simulink model "Channelizer_orig"  (R2026a)
settings: Solver=VariableStepAuto  StopTime=1e-5
InitFcn:
  | init;
values from neighbouring files (symbols this model uses):
  ch0_en = 0    [channelizer_demo_init.m]    (also in init.m)
  ch0_qam = 0    [channelizer_demo_init.m]    (also in init.m)
  ch0_swp = 0    [channelizer_demo_init.m]    (also in init.m)
  ch10_en = 0    [channelizer_demo_init.m]    (also in init.m)
  ch10_qam = 0    [channelizer_demo_init.m]    (also in init.m)
  ch10_swp = 0    [channelizer_demo_init.m]    (also in init.m)
  ch11_en = 0    [channelizer_demo_init.m]    (also in init.m)
  ch11_qam = 0    [channelizer_demo_init.m]    (also in init.m)
  ch11_swp = 0    [channelizer_demo_init.m]    (also in init.m)
  ch12_en = 0    [channelizer_demo_init.m]    (also in init.m)
  ch12_qam = 0    [channelizer_demo_init.m]    (also in init.m)
  ch12_swp = 0    [channelizer_demo_init.m]    (also in init.m)
  ch13_en = 0    [channelizer_demo_init.m]    (also in init.m)
  ch13_qam = 0    [channelizer_demo_init.m]    (also in init.m)
  ch13_swp = 0    [channelizer_demo_init.m]    (also in init.m)
  ch14_en = 0    [channelizer_demo_init.m]    (also in init.m)
  ch14_qam = 0    [channelizer_demo_init.m]    (also in init.m)
  ch14_swp = 0    [channelizer_demo_init.m]    (also in init.m)
  ch15_en = 0    [channelizer_demo_init.m]    (also in init.m)
  ch15_qam = 0    [channelizer_demo_init.m]    (also in init.m)
  ch15_swp = 0    [channelizer_demo_init.m]    (also in init.m)
  ch1_en = 1    [channelizer_demo_init.m]    (also in init.m)
  ch1_qam = 0    [channelizer_demo_init.m]    (also in init.m)
  ch1_swp = 0    [channelizer_demo_init.m]    (also in init.m)
  ch2_en = 1    [channelizer_demo_init.m]    (also in init.m)
  ch2_qam = 0    [channelizer_demo_init.m]    (also in init.m)
  ch2_swp = 0    [channelizer_demo_init.m]    (also in init.m)
  ch3_en = 0    [channelizer_demo_init.m]    (also in init.m)
  ch3_qam = 0    [channelizer_demo_init.m]    (also in init.m)
  ch3_swp = 0    [channelizer_demo_init.m]    (also in init.m)
  ch4_en = 0    [channelizer_demo_init.m]    (also in init.m)
  ch4_qam = 0    [channelizer_demo_init.m]    (also in init.m)
  ch4_swp = 0    [channelizer_demo_init.m]    (also in init.m)
  ch5_en = 1    [channelizer_demo_init.m]    (also in init.m)
  ch5_qam = 1    [channelizer_demo_init.m]    (also in init.m)
  ch5_swp = 0    [channelizer_demo_init.m]    (also in init.m)
  ch6_en = 1    [channelizer_demo_init.m]    (also in init.m)
  ch6_qam = 1    [channelizer_demo_init.m]    (also in init.m)
  ch6_swp = 0    [channelizer_demo_init.m]    (also in init.m)
  ch7_en = 0    [channelizer_demo_init.m]    (also in init.m)
  ch7_qam = 0    [channelizer_demo_init.m]    (also in init.m)
  ch7_swp = 0    [channelizer_demo_init.m]    (also in init.m)
  ch8_en = 0    [channelizer_demo_init.m]    (also in init.m)
  ch8_qam = 0    [channelizer_demo_init.m]    (also in init.m)
  ch8_swp = 0    [channelizer_demo_init.m]    (also in init.m)
  ch9_en = 0    [channelizer_demo_init.m]    (also in init.m)
  ch9_qam = 0    [channelizer_demo_init.m]    (also in init.m)
  ch9_swp = 0    [channelizer_demo_init.m]    (also in init.m)
  ch_filt_coef = 28 * ch_filt_coef / sum(ch_filt_coef(:))    [init.m]
  N = 2*1024    (= 2048)    [hil.m]    (also in init.m = 256)
  nvar = 0.01    [init.m]
  randph = 2*pi*rand(16,1)    [init.m]
  spec1_ch = 1    [channelizer_demo_init.m]    (also in init.m)
  spec2_ch = 2    [channelizer_demo_init.m]    (also in init.m)
  spec3_ch = 5    [channelizer_demo_init.m]    (also in init.m)
  spec4_ch = 6    [channelizer_demo_init.m]    (also in init.m)
  swp_rate0 = 0    [channelizer_demo_init.m]    (also in init.m)
  swp_rate1 = 0    [channelizer_demo_init.m]    (also in init.m)
  swp_rate10 = 0    [channelizer_demo_init.m]    (also in init.m)
  swp_rate11 = 0    [channelizer_demo_init.m]    (also in init.m)
  swp_rate12 = 0    [channelizer_demo_init.m]    (also in init.m)
  swp_rate13 = 0    [channelizer_demo_init.m]    (also in init.m)
  swp_rate14 = 0    [channelizer_demo_init.m]    (also in init.m)
  swp_rate15 = 0    [channelizer_demo_init.m]    (also in init.m)
  swp_rate2 = 0    [channelizer_demo_init.m]    (also in init.m)
  swp_rate3 = 0    [channelizer_demo_init.m]    (also in init.m)
  swp_rate4 = 0    [channelizer_demo_init.m]    (also in init.m)
  swp_rate5 = 0    [channelizer_demo_init.m]    (also in init.m)
  swp_rate6 = 0    [channelizer_demo_init.m]    (also in init.m)
  swp_rate7 = 0    [channelizer_demo_init.m]    (also in init.m)
  swp_rate8 = 0    [channelizer_demo_init.m]    (also in init.m)
  swp_rate9 = 0    [channelizer_demo_init.m]    (also in init.m)
  Ts = 16*(7/4)/8.75e9    (= 3.2e-09)    [init.m]
undefined symbols (not defined in the file or in its folder): Asymmetric, Channelizer, DUT_SSR, jsin, S, vsva2197, xcvc1902
libraries: aieUtilities x20, aieBasic x7, hlsBasic x4, aieDSP x2, vmcUtilities x1
(part 3 of 3)

== system Channelizer_orig/Wideband_Signal/Subsystem5 ==
  swp_en : Inport
  chan_fc : Inport  Port=2
  qam_sym : Inport  Port=3
  qam_en : Inport  Port=4
  chan_en : EnablePort
  Add{1..4} (4 alike) : Sum
  Constant : Constant  Value=complex(ones(28*N,1))  SampleTime=-1
  Constant1 : Constant  Value=complex(zeros(N,27))  VectorParams1D=off  SampleTime=-1
  Constant2 : Constant  Value=(1:28*N)'  SampleTime=-1
  Constant3 : Constant  Value=(1:28*N)'  SampleTime=-1
  Constant4 : Constant  Value=2^32  SampleTime=-1
  Constant5 : Constant  Value=zeros(28*N,1)  SampleTime=-1
  Constant6 : Constant  Value=randph(5)  SampleTime=-1
  Constant7 : Constant  Value=2^32  SampleTime=-1
  Delay1 : Delay  DelayLength=1  InitialCondition=(0:28*N-1)'
  Delay2 : Delay  DelayLength=1  InitialCondition=(1:28*N)'  ExternalReset=Falling  ShowEnablePort=on
      settings: InputPortMap=u0,e6,r5
  Discrete FIR Filter : DiscreteFir  Coefficients=ch_filt_coef  InputProcessing=Columns as channels (frame based)
  Gain1 : Gain  Gain=2*pi  OutDataTypeStr=double
  Gain7 : Gain  Gain=1e-7*swp_rate4  ParamDataTypeStr=double  OutDataTypeStr=double  SaturateOnIntegerOverflow=on
  Gain8 : Gain  Gain=1/16  OutDataTypeStr=double
  Mod : Math  Operator=mod
  Mod1 : Math  Operator=mod
  NOT : Logic  Operator=NOT  IconShape=distinctive  AllPortsSameDT=off  OutDataTypeStr=boolean
  Product : Product
  Product1 : Product
  Product2 : Product
  Reshape : Reshape
  Selector1 : Selector  InputPortWidth=28*N  IndexOptions=Index vector (dialog)  Indices=28*N  OutputSizes=1
  Selector2 : Selector  InputPortWidth=28*N  IndexOptions=Index vector (dialog)  Indices=28*N  OutputSizes=1
  Switch : Switch  Criteria=u2 > Threshold  SaturateOnIntegerOverflow=off  InputSameDT=off
  Switch1 : Switch  Criteria=u2 > Threshold  SaturateOnIntegerOverflow=off  InputSameDT=off
  Transpose : Math  Operator=transpose
  Trigonometric Function : Trigonometry  Operator=cos + jsin
  Vector Concatenate : Concatenate  Mode=Multidimensional array  ConcatenateDimension=2
  chan_out : Outport  OutputWhenDisabled=reset  InitialOutput=zeros(28*N,1)
  wires:
  Product/1 -> chan_out/1
  Switch/1 -> Product/2
  Discrete FIR Filter/1 -> Switch/1
  qam_en/1 -> Switch/2
  Constant/1 -> Switch/3
  Vector Concatenate/1 -> Transpose/1
  qam_sym/1 -> Vector Concatenate/1
  Constant1/1 -> Vector Concatenate/2
  Transpose/1 -> Reshape/1
  Reshape/1 -> Discrete FIR Filter/1
  Delay1/1 -> Product1/1, Selector1/1
  Selector1/1 -> Add3/1
  Constant3/1 -> Add3/2
  Mod/1 -> Delay1/1
  Add3/1 -> Mod/1
  Constant4/1 -> Mod/2
  Constant6/1 -> Add4/1
  Trigonometric Function/1 -> Product/1
  Add4/1 -> Trigonometric Function/1
  chan_fc/1 -> Gain8/1
  Gain8/1 -> Product1/2
  Gain1/1 -> Add4/2
  swp_en/1 -> NOT/1, Delay2/2, Switch1/2
  Constant5/1 -> Switch1/3
  Product2/1 -> Gain7/1
  Gain7/1 -> Switch1/1
  Switch1/1 -> Add1/1
  Product1/1 -> Add1/2
  Add1/1 -> Gain1/1
  Mod1/1 -> Delay2/1
  Constant2/1 -> Add2/2
  Selector2/1 -> Add2/1
  Delay2/1 -> Product2/1, Selector2/1, Product2/2
  Add2/1 -> Mod1/1
  Constant7/1 -> Mod1/2
  NOT/1 -> Delay2/3

== system Channelizer_orig/Wideband_Signal/Subsystem6 ==
  swp_en : Inport
  chan_fc : Inport  Port=2
  qam_sym : Inport  Port=3
  qam_en : Inport  Port=4
  chan_en : EnablePort
  Add{1..4} (4 alike) : Sum
  Constant : Constant  Value=complex(ones(28*N,1))  SampleTime=-1
  Constant1 : Constant  Value=complex(zeros(N,27))  VectorParams1D=off  SampleTime=-1
  Constant2 : Constant  Value=(1:28*N)'  SampleTime=-1
  Constant3 : Constant  Value=(1:28*N)'  SampleTime=-1
  Constant4 : Constant  Value=2^32  SampleTime=-1
  Constant5 : Constant  Value=zeros(28*N,1)  SampleTime=-1
  Constant6 : Constant  Value=randph(6)  SampleTime=-1
  Constant7 : Constant  Value=2^32  SampleTime=-1
  Delay1 : Delay  DelayLength=1  InitialCondition=(0:28*N-1)'
  Delay2 : Delay  DelayLength=1  InitialCondition=(1:28*N)'  ExternalReset=Falling  ShowEnablePort=on
      settings: InputPortMap=u0,e6,r5
  Discrete FIR Filter : DiscreteFir  Coefficients=ch_filt_coef  InputProcessing=Columns as channels (frame based)
  Gain1 : Gain  Gain=2*pi  OutDataTypeStr=double
  Gain7 : Gain  Gain=1e-7*swp_rate5  ParamDataTypeStr=double  OutDataTypeStr=double  SaturateOnIntegerOverflow=on
  Gain8 : Gain  Gain=1/16  OutDataTypeStr=double
  Mod : Math  Operator=mod
  Mod1 : Math  Operator=mod
  NOT : Logic  Operator=NOT  IconShape=distinctive  AllPortsSameDT=off  OutDataTypeStr=boolean
  Product : Product
  Product1 : Product
  Product2 : Product
  Reshape : Reshape
  Selector1 : Selector  InputPortWidth=28*N  IndexOptions=Index vector (dialog)  Indices=28*N  OutputSizes=1
  Selector2 : Selector  InputPortWidth=28*N  IndexOptions=Index vector (dialog)  Indices=28*N  OutputSizes=1
  Switch : Switch  Criteria=u2 > Threshold  SaturateOnIntegerOverflow=off  InputSameDT=off
  Switch1 : Switch  Criteria=u2 > Threshold  SaturateOnIntegerOverflow=off  InputSameDT=off
  Transpose : Math  Operator=transpose
  Trigonometric Function : Trigonometry  Operator=cos + jsin
  Vector Concatenate : Concatenate  Mode=Multidimensional array  ConcatenateDimension=2
  chan_out : Outport  OutputWhenDisabled=reset  InitialOutput=zeros(28*N,1)
  wires:
  Product/1 -> chan_out/1
  Switch/1 -> Product/2
  Discrete FIR Filter/1 -> Switch/1
  qam_en/1 -> Switch/2
  Constant/1 -> Switch/3
  Vector Concatenate/1 -> Transpose/1
  qam_sym/1 -> Vector Concatenate/1
  Constant1/1 -> Vector Concatenate/2
  Transpose/1 -> Reshape/1
  Reshape/1 -> Discrete FIR Filter/1
  Delay1/1 -> Product1/1, Selector1/1
  Selector1/1 -> Add3/1
  Constant3/1 -> Add3/2
  Mod/1 -> Delay1/1
  Add3/1 -> Mod/1
  Constant4/1 -> Mod/2
  Constant6/1 -> Add4/1
  Trigonometric Function/1 -> Product/1
  Add4/1 -> Trigonometric Function/1
  chan_fc/1 -> Gain8/1
  Gain8/1 -> Product1/2
  Gain1/1 -> Add4/2
  swp_en/1 -> NOT/1, Delay2/2, Switch1/2
  Constant5/1 -> Switch1/3
  Product2/1 -> Gain7/1
  Gain7/1 -> Switch1/1
  Switch1/1 -> Add1/1
  Product1/1 -> Add1/2
  Add1/1 -> Gain1/1
  Mod1/1 -> Delay2/1
  Constant2/1 -> Add2/2
  Selector2/1 -> Add2/1
  Delay2/1 -> Product2/1, Selector2/1, Product2/2
  Add2/1 -> Mod1/1
  Constant7/1 -> Mod1/2
  NOT/1 -> Delay2/3

== system Channelizer_orig/Wideband_Signal/Subsystem7 ==
  swp_en : Inport
  chan_fc : Inport  Port=2
  qam_sym : Inport  Port=3
  qam_en : Inport  Port=4
  chan_en : EnablePort
  Add{1..4} (4 alike) : Sum
  Constant : Constant  Value=complex(ones(28*N,1))  SampleTime=-1
  Constant1 : Constant  Value=complex(zeros(N,27))  VectorParams1D=off  SampleTime=-1
  Constant2 : Constant  Value=(1:28*N)'  SampleTime=-1
  Constant3 : Constant  Value=(1:28*N)'  SampleTime=-1
  Constant4 : Constant  Value=2^32  SampleTime=-1
  Constant5 : Constant  Value=zeros(28*N,1)  SampleTime=-1
  Constant6 : Constant  Value=randph(7)  SampleTime=-1
  Constant7 : Constant  Value=2^32  SampleTime=-1
  Delay1 : Delay  DelayLength=1  InitialCondition=(0:28*N-1)'
  Delay2 : Delay  DelayLength=1  InitialCondition=(1:28*N)'  ExternalReset=Falling  ShowEnablePort=on
      settings: InputPortMap=u0,e6,r5
  Discrete FIR Filter : DiscreteFir  Coefficients=ch_filt_coef  InputProcessing=Columns as channels (frame based)
  Gain1 : Gain  Gain=2*pi  OutDataTypeStr=double
  Gain7 : Gain  Gain=1e-7*swp_rate6  ParamDataTypeStr=double  OutDataTypeStr=double  SaturateOnIntegerOverflow=on
  Gain8 : Gain  Gain=1/16  OutDataTypeStr=double
  Mod : Math  Operator=mod
  Mod1 : Math  Operator=mod
  NOT : Logic  Operator=NOT  IconShape=distinctive  AllPortsSameDT=off  OutDataTypeStr=boolean
  Product : Product
  Product1 : Product
  Product2 : Product
  Reshape : Reshape
  Selector1 : Selector  InputPortWidth=28*N  IndexOptions=Index vector (dialog)  Indices=28*N  OutputSizes=1
  Selector2 : Selector  InputPortWidth=28*N  IndexOptions=Index vector (dialog)  Indices=28*N  OutputSizes=1
  Switch : Switch  Criteria=u2 > Threshold  SaturateOnIntegerOverflow=off  InputSameDT=off
  Switch1 : Switch  Criteria=u2 > Threshold  SaturateOnIntegerOverflow=off  InputSameDT=off
  Transpose : Math  Operator=transpose
  Trigonometric Function : Trigonometry  Operator=cos + jsin
  Vector Concatenate : Concatenate  Mode=Multidimensional array  ConcatenateDimension=2
  chan_out : Outport  OutputWhenDisabled=reset  InitialOutput=zeros(28*N,1)
  wires:
  Product/1 -> chan_out/1
  Switch/1 -> Product/2
  Discrete FIR Filter/1 -> Switch/1
  qam_en/1 -> Switch/2
  Constant/1 -> Switch/3
  Vector Concatenate/1 -> Transpose/1
  qam_sym/1 -> Vector Concatenate/1
  Constant1/1 -> Vector Concatenate/2
  Transpose/1 -> Reshape/1
  Reshape/1 -> Discrete FIR Filter/1
  Delay1/1 -> Product1/1, Selector1/1
  Selector1/1 -> Add3/1
  Constant3/1 -> Add3/2
  Mod/1 -> Delay1/1
  Add3/1 -> Mod/1
  Constant4/1 -> Mod/2
  Constant6/1 -> Add4/1
  Trigonometric Function/1 -> Product/1
  Add4/1 -> Trigonometric Function/1
  chan_fc/1 -> Gain8/1
  Gain8/1 -> Product1/2
  Gain1/1 -> Add4/2
  swp_en/1 -> NOT/1, Delay2/2, Switch1/2
  Constant5/1 -> Switch1/3
  Product2/1 -> Gain7/1
  Gain7/1 -> Switch1/1
  Switch1/1 -> Add1/1
  Product1/1 -> Add1/2
  Add1/1 -> Gain1/1
  Mod1/1 -> Delay2/1
  Constant2/1 -> Add2/2
  Selector2/1 -> Add2/1
  Delay2/1 -> Product2/1, Selector2/1, Product2/2
  Add2/1 -> Mod1/1
  Constant7/1 -> Mod1/2
  NOT/1 -> Delay2/3

== system Channelizer_orig/Wideband_Signal/Subsystem8 ==
  swp_en : Inport
  chan_fc : Inport  Port=2
  qam_sym : Inport  Port=3
  qam_en : Inport  Port=4
  chan_en : EnablePort
  Add{1..4} (4 alike) : Sum
  Constant : Constant  Value=complex(ones(28*N,1))  SampleTime=-1
  Constant1 : Constant  Value=complex(zeros(N,27))  VectorParams1D=off  SampleTime=-1
  Constant2 : Constant  Value=(1:28*N)'  SampleTime=-1
  Constant3 : Constant  Value=(1:28*N)'  SampleTime=-1
  Constant4 : Constant  Value=2^32  SampleTime=-1
  Constant5 : Constant  Value=zeros(28*N,1)  SampleTime=-1
  Constant6 : Constant  Value=randph(8)  SampleTime=-1
  Constant7 : Constant  Value=2^32  SampleTime=-1
  Delay1 : Delay  DelayLength=1  InitialCondition=(0:28*N-1)'
  Delay2 : Delay  DelayLength=1  InitialCondition=(1:28*N)'  ExternalReset=Falling  ShowEnablePort=on
      settings: InputPortMap=u0,e6,r5
  Discrete FIR Filter : DiscreteFir  Coefficients=ch_filt_coef  InputProcessing=Columns as channels (frame based)
  Gain1 : Gain  Gain=2*pi  OutDataTypeStr=double
  Gain7 : Gain  Gain=1e-7*swp_rate7  ParamDataTypeStr=double  OutDataTypeStr=double  SaturateOnIntegerOverflow=on
  Gain8 : Gain  Gain=1/16  OutDataTypeStr=double
  Mod : Math  Operator=mod
  Mod1 : Math  Operator=mod
  NOT : Logic  Operator=NOT  IconShape=distinctive  AllPortsSameDT=off  OutDataTypeStr=boolean
  Product : Product
  Product1 : Product
  Product2 : Product
  Reshape : Reshape
  Selector1 : Selector  InputPortWidth=28*N  IndexOptions=Index vector (dialog)  Indices=28*N  OutputSizes=1
  Selector2 : Selector  InputPortWidth=28*N  IndexOptions=Index vector (dialog)  Indices=28*N  OutputSizes=1
  Switch : Switch  Criteria=u2 > Threshold  SaturateOnIntegerOverflow=off  InputSameDT=off
  Switch1 : Switch  Criteria=u2 > Threshold  SaturateOnIntegerOverflow=off  InputSameDT=off
  Transpose : Math  Operator=transpose
  Trigonometric Function : Trigonometry  Operator=cos + jsin
  Vector Concatenate : Concatenate  Mode=Multidimensional array  ConcatenateDimension=2
  chan_out : Outport  OutputWhenDisabled=reset  InitialOutput=zeros(28*N,1)
  wires:
  Product/1 -> chan_out/1
  Switch/1 -> Product/2
  Discrete FIR Filter/1 -> Switch/1
  qam_en/1 -> Switch/2
  Constant/1 -> Switch/3
  Vector Concatenate/1 -> Transpose/1
  qam_sym/1 -> Vector Concatenate/1
  Constant1/1 -> Vector Concatenate/2
  Transpose/1 -> Reshape/1
  Reshape/1 -> Discrete FIR Filter/1
  Delay1/1 -> Product1/1, Selector1/1
  Selector1/1 -> Add3/1
  Constant3/1 -> Add3/2
  Mod/1 -> Delay1/1
  Add3/1 -> Mod/1
  Constant4/1 -> Mod/2
  Constant6/1 -> Add4/1
  Trigonometric Function/1 -> Product/1
  Add4/1 -> Trigonometric Function/1
  chan_fc/1 -> Gain8/1
  Gain8/1 -> Product1/2
  Gain1/1 -> Add4/2
  swp_en/1 -> NOT/1, Delay2/2, Switch1/2
  Constant5/1 -> Switch1/3
  Product2/1 -> Gain7/1
  Gain7/1 -> Switch1/1
  Switch1/1 -> Add1/1
  Product1/1 -> Add1/2
  Add1/1 -> Gain1/1
  Mod1/1 -> Delay2/1
  Constant2/1 -> Add2/2
  Selector2/1 -> Add2/1
  Delay2/1 -> Product2/1, Selector2/1, Product2/2
  Add2/1 -> Mod1/1
  Constant7/1 -> Mod1/2
  NOT/1 -> Delay2/3

== system Channelizer_orig/Wideband_Signal/Subsystem9 ==
  swp_en : Inport
  chan_fc : Inport  Port=2
  qam_sym : Inport  Port=3
  qam_en : Inport  Port=4
  chan_en : EnablePort
  Add{1..4} (4 alike) : Sum
  Constant : Constant  Value=complex(ones(28*N,1))  SampleTime=-1
  Constant1 : Constant  Value=complex(zeros(N,27))  VectorParams1D=off  SampleTime=-1
  Constant2 : Constant  Value=(1:28*N)'  SampleTime=-1
  Constant3 : Constant  Value=(1:28*N)'  SampleTime=-1
  Constant4 : Constant  Value=2^32  SampleTime=-1
  Constant5 : Constant  Value=zeros(28*N,1)  SampleTime=-1
  Constant6 : Constant  Value=randph(9)  SampleTime=-1
  Constant7 : Constant  Value=2^32  SampleTime=-1
  Delay1 : Delay  DelayLength=1  InitialCondition=(0:28*N-1)'
  Delay2 : Delay  DelayLength=1  InitialCondition=(1:28*N)'  ExternalReset=Falling  ShowEnablePort=on
      settings: InputPortMap=u0,e6,r5
  Discrete FIR Filter : DiscreteFir  Coefficients=ch_filt_coef  InputProcessing=Columns as channels (frame based)
  Gain1 : Gain  Gain=2*pi  OutDataTypeStr=double
  Gain7 : Gain  Gain=1e-7*swp_rate8  ParamDataTypeStr=double  OutDataTypeStr=double  SaturateOnIntegerOverflow=on
  Gain8 : Gain  Gain=1/16  OutDataTypeStr=double
  Mod : Math  Operator=mod
  Mod1 : Math  Operator=mod
  NOT : Logic  Operator=NOT  IconShape=distinctive  AllPortsSameDT=off  OutDataTypeStr=boolean
  Product : Product
  Product1 : Product
  Product2 : Product
  Reshape : Reshape
  Selector1 : Selector  InputPortWidth=28*N  IndexOptions=Index vector (dialog)  Indices=28*N  OutputSizes=1
  Selector2 : Selector  InputPortWidth=28*N  IndexOptions=Index vector (dialog)  Indices=28*N  OutputSizes=1
  Switch : Switch  Criteria=u2 > Threshold  SaturateOnIntegerOverflow=off  InputSameDT=off
  Switch1 : Switch  Criteria=u2 > Threshold  SaturateOnIntegerOverflow=off  InputSameDT=off
  Transpose : Math  Operator=transpose
  Trigonometric Function : Trigonometry  Operator=cos + jsin
  Vector Concatenate : Concatenate  Mode=Multidimensional array  ConcatenateDimension=2
  chan_out : Outport  OutputWhenDisabled=reset  InitialOutput=zeros(28*N,1)
  wires:
  Product/1 -> chan_out/1
  Switch/1 -> Product/2
  Discrete FIR Filter/1 -> Switch/1
  qam_en/1 -> Switch/2
  Constant/1 -> Switch/3
  Vector Concatenate/1 -> Transpose/1
  qam_sym/1 -> Vector Concatenate/1
  Constant1/1 -> Vector Concatenate/2
  Transpose/1 -> Reshape/1
  Reshape/1 -> Discrete FIR Filter/1
  Delay1/1 -> Product1/1, Selector1/1
  Selector1/1 -> Add3/1
  Constant3/1 -> Add3/2
  Mod/1 -> Delay1/1
  Add3/1 -> Mod/1
  Constant4/1 -> Mod/2
  Constant6/1 -> Add4/1
  Trigonometric Function/1 -> Product/1
  Add4/1 -> Trigonometric Function/1
  chan_fc/1 -> Gain8/1
  Gain8/1 -> Product1/2
  Gain1/1 -> Add4/2
  swp_en/1 -> NOT/1, Delay2/2, Switch1/2
  Constant5/1 -> Switch1/3
  Product2/1 -> Gain7/1
  Gain7/1 -> Switch1/1
  Switch1/1 -> Add1/1
  Product1/1 -> Add1/2
  Add1/1 -> Gain1/1
  Mod1/1 -> Delay2/1
  Constant2/1 -> Add2/2
  Selector2/1 -> Add2/1
  Delay2/1 -> Product2/1, Selector2/1, Product2/2
  Add2/1 -> Mod1/1
  Constant7/1 -> Mod1/2
  NOT/1 -> Delay2/3
